simulink model "frt_only_up"  (R2012b)
settings: Solver=FixedStepDiscrete  SolverMode=SingleTasking  StartTime=0.0  StopTime=10000  RelTol=1e-3
undefined symbols (not defined in the file or in its folder): Down, Up
libraries: xbsIndex_r4 x5535, casper_library_misc x12, casper_library_communications x8, casper_library_scopes x2, xps_library x1
(part 8 of 48)

== system frt_only_up/trig1 ==
  synci : Inport
  adc_data : Inport  Port=2
  trig_pnt : Inport  Port=3
  Delay1 : xbsIndex_r4/Delay  rst=off  infoeditControl=Selection of Reset will increase slice count due to use of real FFs and instead of SRLs  en=off  latency=mult_latency+2  dbl_ovrd=off  reg_retiming=on  block_type=delay
      settings: block_version=11.4
  Delay2 : xbsIndex_r4/Delay  rst=off  infoeditControl=Selection of Reset will increase slice count due to use of real FFs and instead of SRLs  en=off  latency=mult_latency+2  dbl_ovrd=off  reg_retiming=on  block_type=delay
      settings: block_version=11.4
  Logical1 : xbsIndex_r4/Logical  logical_function=OR  inputs=4  en=off  latency=1  precision=Full  arith_type=Unsigned  n_bits=16  bin_pt=0  align_bp=on  dbl_ovrd=off  block_type=logical
  Mult : xbsIndex_r4/Mult  precision=Full  arith_type=Unsigned  n_bits=16  bin_pt=14  quantization=Truncate  overflow=Saturate  en=off  latency=mult_latency  dbl_ovrd=off  use_behavioral_HDL=on  opt=Speed  use_embedded=on  optimum_pipeline=off  pipeline=on  use_rpm=on  placement_style=Rectangular shape  block_type=mult
      settings: xl_area=[0, 0, 0, 0, 0, 0, 0]  block_version=10.1.3
  Reinterpret4 : xbsIndex_r4/Reinterpret  force_arith_type=on  arith_type="Signed  (2's comp)"  force_bin_pt=on  bin_pt=9  block_type=reinterpret
      settings: block_version=10.1.3
  Slice3 : xbsIndex_r4/Slice  nbits=10  boolean_output=off  mode=Lower Bit Location + Width  bit1=0  base1=MSB of Input  bit0=0  base0=LSB of Input  dbl_ovrd=off  block_type=slice
      settings: block_version=10.1.3
  Subsystem1 : Subsystem  mask{mult_latency=mult_latency}
      mask prompts: mult_latency "Multiplier latency"
  Subsystem2 : Subsystem  mask{mult_latency=mult_latency}
      mask prompts: mult_latency "Multiplier latency"
  Subsystem3 : Subsystem  mask{mult_latency=mult_latency}
      mask prompts: mult_latency "Multiplier latency"
  Subsystem5 : Subsystem  mask{mult_latency=mult_latency}
      mask prompts: mult_latency "Multiplier latency"
  bus_expand : Subsystem  AncestorBlock=casper_library_flow_control/bus_expand  mask(bus_expand){mode=divisions of equal size, outputNum=4, outputWidth=10, outputBinaryPt=9, outputArithmeticType=1, show_format=off, outputToWorkspace=off, variablePrefix=out, outputToModelAsWell=on}
      mask prompts: outputNum "Number of outputs:"; outputWidth "Output width:"; outputBinaryPt "Output binary point position:"; outputArithmeticType "Output arithmetic type (ufix=0, fix=1, bool=2):"; show_format "Print format string?"; outputToWorkspace "Output to workspace?"; variablePrefix "Variable name prefix:"; outputToModelAsWell "Output to model as well?"
      mask help:
      | Expands a 'bus' made using a bus_create or Xilinx
      | concat block.
      | The input will be divided into the specified number
      | of outputs with the specified arithmetic types.
      | Divisions are made from most significant bit.
      mask init: same as frt_only_up/bus_expand2
      settings: AttributesFormatString=4 outputs
      mask TypeOptions mode: divisions of equal size | divisions of arbitrary size
      mask Callback mode: bus_expand_callback();
      mask Callback outputWidth: bus_expand_callback();
      mask Callback outputToWorkspace: bus_expand_callback();
  synco : Outport
  data : Outport  Port=2
  trig : Outport  Port=3
  wires:
  bus_expand/4(lsb_out1) -> Subsystem3/1(din)
  bus_expand/3(out2) -> Subsystem2/1(din)
  bus_expand/2(out3) -> Subsystem1/1(din)
  bus_expand/1(msb_out4) -> Subsystem5/1(din)
  Delay1/1 -> data/1
  trig_pnt/1 -> Slice3/1
  Slice3/1 -> Reinterpret4/1
  Reinterpret4/1 -> Mult/2, Mult/1
  Mult/1 -> Subsystem3/2(thresh), Subsystem2/2(thresh), Subsystem1/2(thresh), Subsystem5/2(thresh)
  Logical1/1 -> trig/1
  adc_data/1 -> bus_expand/1(bus_in), Delay1/1
  Subsystem3/1(trig) -> Logical1/4
  Subsystem2/1(trig) -> Logical1/3
  Subsystem1/1(trig) -> Logical1/2
  Subsystem5/1(trig) -> Logical1/1
  synci/1 -> Delay2/1
  Delay2/1 -> synco/1

== system frt_only_up/trigger_level ==
  sim_1 : Inport
  frt_only_up_trigger_level_user_data_out : xbsIndex_r4/Gateway In  gui_display_data_type=Fixed-point  arith_type=Unsigned  n_bits=32  bin_pt=0  preci_type=Single  exp_width=8  frac_width=24  quantization="Round  (unbiased: +/- Inf)"  overflow=Saturate  period=1  dbl_ovrd=off  timing_constraint=None  locs_specified=off  LOCs={}  UseAsADC=off  ADCChannel='1'  inherit_from_input=off  hdl_port=on  block_type=gatewayin
  io_delay : xbsIndex_r4/Delay  rst=off  infoeditControl=Selection of Reset will increase slice count due to use of real FFs and instead of SRLs  en=off  latency=0  dbl_ovrd=off  reg_retiming=on  block_type=delay
  reint1 : xbsIndex_r4/Reinterpret  force_arith_type=on  arith_type=Unsigned  force_bin_pt=on  bin_pt=0  block_type=reinterpret
  slice_trigger_level : xbsIndex_r4/Slice  nbits=32  boolean_output=off  mode=Lower Bit Location + Width  bit1=0  base1=MSB of Input  bit0=0  base0=LSB of Input  dbl_ovrd=off  block_type=slice
  in_trigger_level : Outport
  wires:
  frt_only_up_trigger_level_user_data_out/1 -> io_delay/1
  sim_1/1 -> frt_only_up_trigger_level_user_data_out/1
  io_delay/1 -> slice_trigger_level/1
  slice_trigger_level/1 -> reint1/1
  reint1/1 -> in_trigger_level/1

== system frt_only_up/tx_metadata ==
  sim_1 : Inport
  sim_2 : Inport  Port=2
  convert1_1 : DataTypeConversion  OutDataTypeStr=fixdt('ufix16_En0')  LockScale=on
  convert1_2 : DataTypeConversion  OutDataTypeStr=fixdt('ufix16_En0')  LockScale=on
  convert2_1 : DataTypeConversion  OutDataTypeStr=fixdt('ufix16_En0')  ConvertRealWorld=Stored Integer (SI)  LockScale=on
  convert2_2 : DataTypeConversion  OutDataTypeStr=fixdt('ufix16_En0')  ConvertRealWorld=Stored Integer (SI)  LockScale=on
  frt_only_up_tx_metadata_user_data_out : xbsIndex_r4/Gateway In  gui_display_data_type=Fixed-point  arith_type=Unsigned  n_bits=32  bin_pt=0  preci_type=Single  exp_width=8  frac_width=24  quantization="Round  (unbiased: +/- Inf)"  overflow=Saturate  period=1  dbl_ovrd=off  timing_constraint=None  locs_specified=off  LOCs={}  UseAsADC=off  ADCChannel='1'  inherit_from_input=off  hdl_port=on  block_type=gatewayin
  gain_1 : Gain  Gain=65536
  gain_2 : Gain
  io_delay : xbsIndex_r4/Delay  rst=off  infoeditControl=Selection of Reset will increase slice count due to use of real FFs and instead of SRLs  en=off  latency=0  dbl_ovrd=off  reg_retiming=on  block_type=delay
  reint1 : xbsIndex_r4/Reinterpret  force_arith_type=on  arith_type=Unsigned  force_bin_pt=on  bin_pt=0  block_type=reinterpret
  reint2 : xbsIndex_r4/Reinterpret  force_arith_type=on  arith_type=Unsigned  force_bin_pt=on  bin_pt=0  block_type=reinterpret
  sim_add : Sum  OutDataTypeStr=uint32
  slice_board_id : xbsIndex_r4/Slice  nbits=16  boolean_output=off  mode=Lower Bit Location + Width  bit1=0  base1=MSB of Input  bit0=0  base0=LSB of Input  dbl_ovrd=off  block_type=slice
  slice_porttx : xbsIndex_r4/Slice  nbits=16  boolean_output=off  mode=Lower Bit Location + Width  bit1=0  base1=MSB of Input  bit0=16  base0=LSB of Input  dbl_ovrd=off  block_type=slice
  in_porttx : Outport
  in_board_id : Outport  Port=2
  wires:
  frt_only_up_tx_metadata_user_data_out/1 -> io_delay/1
  sim_add/1 -> frt_only_up_tx_metadata_user_data_out/1
  sim_1/1 -> convert1_1/1
  convert1_1/1 -> convert2_1/1
  convert2_1/1 -> gain_1/1
  gain_1/1 -> sim_add/1
  io_delay/1 -> slice_porttx/1, slice_board_id/1
  slice_porttx/1 -> reint1/1
  reint1/1 -> in_porttx/1
  sim_2/1 -> convert1_2/1
  convert1_2/1 -> convert2_2/1
  convert2_2/1 -> gain_2/1
  gain_2/1 -> sim_add/2
  slice_board_id/1 -> reint2/1
  reint2/1 -> in_board_id/1

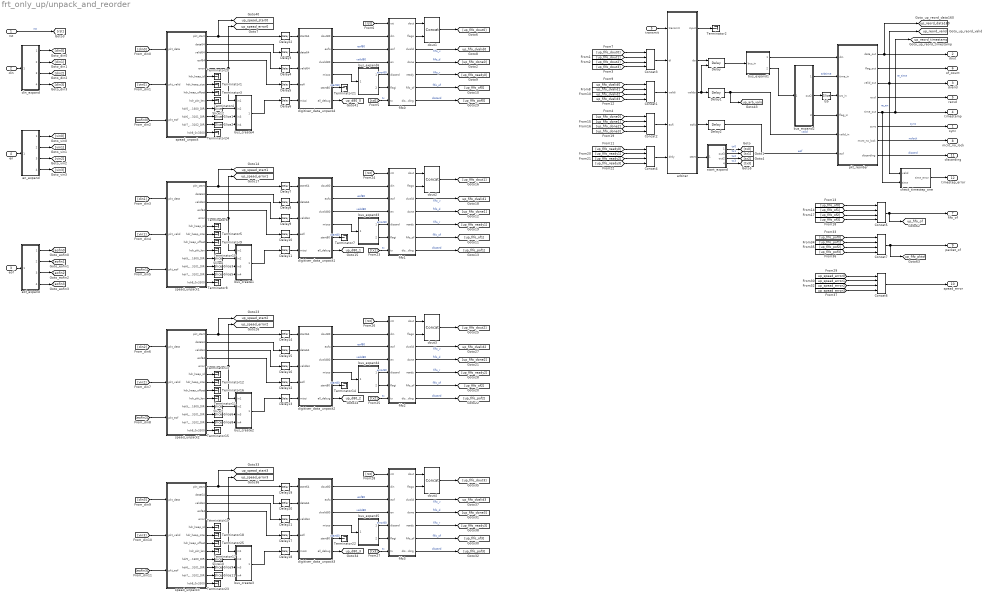
== system frt_only_up/unpack_and_reorder ==
  rst : Inport
  din : Inport  Port=2
  eof : Inport  Port=3
  en : Inport  Port=4
  transmit : Inport  Port=5
  Concat{1..7} (7 alike) : xbsIndex_r4/Concat  num_inputs=4  dbl_ovrd=off  block_type=concat
  Delay : xbsIndex_r4/Delay  rst=off  infoeditControl=Selection of Reset will increase slice count due to use of real FFs and instead of SRLs  en=on  latency=1  dbl_ovrd=off  reg_retiming=on  block_type=delay
  Delay{1..22} (22 alike) : xbsIndex_r4/Delay  rst=off  infoeditControl=Selection of Reset will increase slice count due to use of real FFs and instead of SRLs  en=off  latency=1  dbl_ovrd=off  reg_retiming=on  block_type=delay
      Delay10 settings: block_version=11.4
      Delay11 settings: block_version=11.4
      Delay12 settings: block_version=11.4
      Delay13 settings: block_version=11.4
      Delay14 settings: block_version=11.4
      Delay15 settings: block_version=11.4
      Delay16 settings: block_version=11.4
      Delay17 settings: block_version=11.4
      Delay18 settings: block_version=11.4
      Delay19 settings: block_version=11.4
      Delay20 settings: block_version=11.4
      Delay21 settings: block_version=11.4
      Delay22 settings: block_version=11.4
      Delay3 settings: block_version=11.4
      Delay4 settings: block_version=11.4
      Delay5 settings: block_version=11.4
      Delay6 settings: block_version=11.4
      Delay7 settings: block_version=11.4
      Delay8 settings: block_version=11.4
      Delay9 settings: block_version=11.4
  Slice{1,3,6,9} (4 alike) : xbsIndex_r4/Slice  nbits=2  boolean_output=off  mode=Lower Bit Location + Width  bit1=0  base1=MSB of Input  bit0=0  base0=LSB of Input  dbl_ovrd=off  block_type=slice
  Slice{4,7,10,12} (4 alike) : xbsIndex_r4/Slice  nbits=48 - n_bits_timestep  boolean_output=off  mode=Upper Bit Location + Width  bit1=0  base1=MSB of Input  bit0=0  base0=LSB of Input  dbl_ovrd=off  block_type=slice
  Slice{2,5,8,11} (4 alike) : xbsIndex_r4/Slice  nbits=1  boolean_output=off  mode=Lower Bit Location + Width  bit1=0  base1=MSB of Input  bit0=0  base0=LSB of Input  dbl_ovrd=off  block_type=slice
  Terminator{1..25} (25 alike) : Terminator
  arbiter : Subsystem  mask{n_inputs=4, n_bits_input=160 + 48 - n_bits_timestep + 2 + 1, mux_latency=1}
      mask prompts: n_inputs "number of inputs"; n_bits_input "input bit widths"; mux_latency "mux latency"
      mask init:
      | set_param([gcb, '/eofi_mux'], ...
      |     'n_bits', 'ones(1, n_inputs)', ...
      |     'mux_latency', 'mux_latency', ...
      |     'cmplx', 'off', 'misc', 'off');
      | set_param([gcb, '/di_mux'], ...
      |     'n_bits', 'repmat(n_bits_input, 1, n_inputs)', ...
      |     'mux_latency', 'mux_latency', ...
      |     'cmplx', 'off', 'misc', 'off');
      | set_param([gcb, '/validi_mux'], ...
      |     'n_bits', 'ones(1, n_inputs)', ...
      |     'mux_latency', 'mux_latency', ...
      |     'cmplx', 'off', 'misc', 'off');
      | set_param([gcb, '/busy_edge_rep'], ...
      |     'replication', 'n_inputs', ...
      |     'misc', 'off');
  bus_create1 : Subsystem  AncestorBlock=casper_library_flow_control/bus_create  mask(bus_create){inputNum=4}
      mask prompts: inputNum "Number of inputs:"
      mask init:
      | bus_create_init(gcb,...
      |     'inputNum', inputNum);
  bus_create2 : Subsystem  AncestorBlock=casper_library_flow_control/bus_create  mask(bus_create){inputNum=4}
      mask prompts: inputNum "Number of inputs:"
      mask init:
      | bus_create_init(gcb,...
      |     'inputNum', inputNum);
  bus_create3 : Subsystem  AncestorBlock=casper_library_flow_control/bus_create  mask(bus_create){inputNum=4}
      mask prompts: inputNum "Number of inputs:"
      mask init:
      | bus_create_init(gcb,...
      |     'inputNum', inputNum);
  bus_create4 : Subsystem  AncestorBlock=casper_library_flow_control/bus_create  mask(bus_create){inputNum=4}
      mask prompts: inputNum "Number of inputs:"
      mask init:
      | bus_create_init(gcb,...
      |     'inputNum', inputNum);
  bus_expand1 : Subsystem  AncestorBlock=casper_library_flow_control/bus_expand  mask(bus_expand){mode=divisions of arbitrary size, outputNum=1, outputWidth=[160, sum([48 - n_bits_timestep, 2, 1])], outputBinaryPt=[0 0], outputArithmeticType=[0 0], show_format=off, outputToWorkspace=off, variablePrefix=out, outputToModelAsWell=on}
      mask prompts: outputNum "Number of outputs:"; outputWidth "Output width [msb ... lsb]:"; outputBinaryPt "Output binary point position [msb ... lsb]:"; outputArithmeticType "Output arithmetic type (ufix=0, fix=1, bool=2) [msb ... lsb]:"; show_format "Print format string?"; outputToWorkspace "Output to workspace?"; variablePrefix "Variable name prefix:"; outputToModelAsWell "Output to model as well?"
      mask help:
      | Expands a 'bus' made using a bus_create or Xilinx
      | concat block.
      | The input will be divided into the specified number
      | of outputs with the specified arithmetic types.
      | Divisions are made from most significant bit.
      mask init: same as frt_only_up/bus_expand2
      settings: AttributesFormatString=2 outputs
      mask TypeOptions mode: divisions of equal size | divisions of arbitrary size
      mask Callback mode: bus_expand_callback();
      mask Callback outputWidth: bus_expand_callback();
      mask Callback outputToWorkspace: bus_expand_callback();
  bus_expand2 : Subsystem  AncestorBlock=casper_library_flow_control/bus_expand  mask(bus_expand){mode=divisions of arbitrary size, outputNum=1, outputWidth=[48 - n_bits_timestep, 2, 1], outputBinaryPt=[0 0 0], outputArithmeticType=[0 0 0], show_format=off, outputToWorkspace=off, variablePrefix=out, outputToModelAsWell=on}
      mask prompts: outputNum "Number of outputs:"; outputWidth "Output width [msb ... lsb]:"; outputBinaryPt "Output binary point position [msb ... lsb]:"; outputArithmeticType "Output arithmetic type (ufix=0, fix=1, bool=2) [msb ... lsb]:"; show_format "Print format string?"; outputToWorkspace "Output to workspace?"; variablePrefix "Variable name prefix:"; outputToModelAsWell "Output to model as well?"
      mask help:
      | Expands a 'bus' made using a bus_create or Xilinx
      | concat block.
      | The input will be divided into the specified number
      | of outputs with the specified arithmetic types.
      | Divisions are made from most significant bit.
      mask init: same as frt_only_up/bus_expand2
      settings: AttributesFormatString=3 outputs
      mask TypeOptions mode: divisions of equal size | divisions of arbitrary size
      mask Callback mode: bus_expand_callback();
      mask Callback outputWidth: bus_expand_callback();
      mask Callback outputToWorkspace: bus_expand_callback();
  bus_expand3 : Subsystem  AncestorBlock=casper_library_flow_control/bus_expand  mask(bus_expand){mode=divisions of arbitrary size, outputNum=1, outputWidth=[1, sum([48 - n_bits_timestep, 2, 1])], outputBinaryPt=[0 0], outputArithmeticType=[2 0], show_format=off, outputToWorkspace=off, variablePrefix=out, outputToModelAsWell=on}
      mask prompts: outputNum "Number of outputs:"; outputWidth "Output width [msb ... lsb]:"; outputBinaryPt "Output binary point position [msb ... lsb]:"; outputArithmeticType "Output arithmetic type (ufix=0, fix=1, bool=2) [msb ... lsb]:"; show_format "Print format string?"; outputToWorkspace "Output to workspace?"; variablePrefix "Variable name prefix:"; outputToModelAsWell "Output to model as well?"
      mask help:
      | Expands a 'bus' made using a bus_create or Xilinx
      | concat block.
      | The input will be divided into the specified number
      | of outputs with the specified arithmetic types.
      | Divisions are made from most significant bit.
      mask init: same as frt_only_up/bus_expand2
      settings: AttributesFormatString=2 outputs
      mask TypeOptions mode: divisions of equal size | divisions of arbitrary size
      mask Callback mode: bus_expand_callback();
      mask Callback outputWidth: bus_expand_callback();
      mask Callback outputToWorkspace: bus_expand_callback();
  bus_expand4 : Subsystem  AncestorBlock=casper_library_flow_control/bus_expand  mask(bus_expand){mode=divisions of arbitrary size, outputNum=1, outputWidth=[1, sum([48 - n_bits_timestep, 2, 1])], outputBinaryPt=[0 0], outputArithmeticType=[2 0], show_format=off, outputToWorkspace=off, variablePrefix=out, outputToModelAsWell=on}
      mask prompts: outputNum "Number of outputs:"; outputWidth "Output width [msb ... lsb]:"; outputBinaryPt "Output binary point position [msb ... lsb]:"; outputArithmeticType "Output arithmetic type (ufix=0, fix=1, bool=2) [msb ... lsb]:"; show_format "Print format string?"; outputToWorkspace "Output to workspace?"; variablePrefix "Variable name prefix:"; outputToModelAsWell "Output to model as well?"
      mask help:
      | Expands a 'bus' made using a bus_create or Xilinx
      | concat block.
      | The input will be divided into the specified number
      | of outputs with the specified arithmetic types.
      | Divisions are made from most significant bit.
      mask init: same as frt_only_up/bus_expand2
      settings: AttributesFormatString=2 outputs
      mask TypeOptions mode: divisions of equal size | divisions of arbitrary size
      mask Callback mode: bus_expand_callback();
      mask Callback outputWidth: bus_expand_callback();
      mask Callback outputToWorkspace: bus_expand_callback();
  bus_expand5 : Subsystem  AncestorBlock=casper_library_flow_control/bus_expand  mask(bus_expand){mode=divisions of arbitrary size, outputNum=1, outputWidth=[1, sum([48 - n_bits_timestep, 2, 1])], outputBinaryPt=[0 0], outputArithmeticType=[2 0], show_format=off, outputToWorkspace=off, variablePrefix=out, outputToModelAsWell=on}
      mask prompts: outputNum "Number of outputs:"; outputWidth "Output width [msb ... lsb]:"; outputBinaryPt "Output binary point position [msb ... lsb]:"; outputArithmeticType "Output arithmetic type (ufix=0, fix=1, bool=2) [msb ... lsb]:"; show_format "Print format string?"; outputToWorkspace "Output to workspace?"; variablePrefix "Variable name prefix:"; outputToModelAsWell "Output to model as well?"
      mask help:
      | Expands a 'bus' made using a bus_create or Xilinx
      | concat block.
      | The input will be divided into the specified number
      | of outputs with the specified arithmetic types.
      | Divisions are made from most significant bit.
      mask init: same as frt_only_up/bus_expand2
      settings: AttributesFormatString=2 outputs
      mask TypeOptions mode: divisions of equal size | divisions of arbitrary size
      mask Callback mode: bus_expand_callback();
      mask Callback outputWidth: bus_expand_callback();
      mask Callback outputToWorkspace: bus_expand_callback();
  bus_expand6 : Subsystem  AncestorBlock=casper_library_flow_control/bus_expand  mask(bus_expand){mode=divisions of arbitrary size, outputNum=1, outputWidth=[1, sum([48 - n_bits_timestep, 2, 1])], outputBinaryPt=[0 0], outputArithmeticType=[2 0], show_format=off, outputToWorkspace=off, variablePrefix=out, outputToModelAsWell=on}
      mask prompts: outputNum "Number of outputs:"; outputWidth "Output width [msb ... lsb]:"; outputBinaryPt "Output binary point position [msb ... lsb]:"; outputArithmeticType "Output arithmetic type (ufix=0, fix=1, bool=2) [msb ... lsb]:"; show_format "Print format string?"; outputToWorkspace "Output to workspace?"; variablePrefix "Variable name prefix:"; outputToModelAsWell "Output to model as well?"
      mask help:
      | Expands a 'bus' made using a bus_create or Xilinx
      | concat block.
      | The input will be divided into the specified number
      | of outputs with the specified arithmetic types.
      | Divisions are made from most significant bit.
      mask init: same as frt_only_up/bus_expand2
      settings: AttributesFormatString=2 outputs
      mask TypeOptions mode: divisions of equal size | divisions of arbitrary size
      mask Callback mode: bus_expand_callback();
      mask Callback outputWidth: bus_expand_callback();
      mask Callback outputToWorkspace: bus_expand_callback();
  check_timestep_one : Subsystem
  digitiser_data_unpack1 : Subsystem
  digitiser_data_unpack2 : Subsystem
  digitiser_data_unpack3 : Subsystem
  digitiser_data_unpack4 : Subsystem
  din_expand : Subsystem  AncestorBlock=casper_library_flow_control/bus_expand  mask(bus_expand){mode=divisions of equal size, outputNum=4, outputWidth=64, outputBinaryPt=0, outputArithmeticType=0, show_format=off, outputToWorkspace=off, variablePrefix=out, outputToModelAsWell=on}
      mask prompts: outputNum "Number of outputs:"; outputWidth "Output width:"; outputBinaryPt "Output binary point position:"; outputArithmeticType "Output arithmetic type (ufix=0, fix=1, bool=2):"; show_format "Print format string?"; outputToWorkspace "Output to workspace?"; variablePrefix "Variable name prefix:"; outputToModelAsWell "Output to model as well?"
      mask help:
      | Expands a 'bus' made using a bus_create or Xilinx
      | concat block.
      | The input will be divided into the specified number
      | of outputs with the specified arithmetic types.
      | Divisions are made from most significant bit.
      mask init: same as frt_only_up/bus_expand2
      settings: AttributesFormatString=4 outputs
      mask TypeOptions mode: divisions of equal size | divisions of arbitrary size
      mask Callback mode: bus_expand_callback();
      mask Callback outputWidth: bus_expand_callback();
      mask Callback outputToWorkspace: bus_expand_callback();
  dout{1..4} (4 alike) : xbsIndex_r4/Concat  num_inputs=2  dbl_ovrd=off  block_type=concat
  en_expand : Subsystem  AncestorBlock=casper_library_flow_control/bus_expand  mask(bus_expand){mode=divisions of equal size, outputNum=4, outputWidth=1, outputBinaryPt=0, outputArithmeticType=2, show_format=off, outputToWorkspace=off, variablePrefix=out, outputToModelAsWell=on}
      mask prompts: outputNum "Number of outputs:"; outputWidth "Output width:"; outputBinaryPt "Output binary point position:"; outputArithmeticType "Output arithmetic type (ufix=0, fix=1, bool=2):"; show_format "Print format string?"; outputToWorkspace "Output to workspace?"; variablePrefix "Variable name prefix:"; outputToModelAsWell "Output to model as well?"
      mask help:
      | Expands a 'bus' made using a bus_create or Xilinx
      | concat block.
      | The input will be divided into the specified number
      | of outputs with the specified arithmetic types.
      | Divisions are made from most significant bit.
      mask init: same as frt_only_up/bus_expand2
      settings: AttributesFormatString=4 outputs
      mask TypeOptions mode: divisions of equal size | divisions of arbitrary size
      mask Callback mode: bus_expand_callback();
      mask Callback outputWidth: bus_expand_callback();
      mask Callback outputToWorkspace: bus_expand_callback();
  eof_expand : Subsystem  AncestorBlock=casper_library_flow_control/bus_expand  mask(bus_expand){mode=divisions of equal size, outputNum=4, outputWidth=1, outputBinaryPt=0, outputArithmeticType=2, show_format=off, outputToWorkspace=off, variablePrefix=out, outputToModelAsWell=on}
      mask prompts: outputNum "Number of outputs:"; outputWidth "Output width:"; outputBinaryPt "Output binary point position:"; outputArithmeticType "Output arithmetic type (ufix=0, fix=1, bool=2):"; show_format "Print format string?"; outputToWorkspace "Output to workspace?"; variablePrefix "Variable name prefix:"; outputToModelAsWell "Output to model as well?"
      mask help:
      | Expands a 'bus' made using a bus_create or Xilinx
      | concat block.
      | The input will be divided into the specified number
      | of outputs with the specified arithmetic types.
      | Divisions are made from most significant bit.
      mask init: same as frt_only_up/bus_expand2
      settings: AttributesFormatString=4 outputs
      mask TypeOptions mode: divisions of equal size | divisions of arbitrary size
      mask Callback mode: bus_expand_callback();
      mask Callback outputWidth: bus_expand_callback();
      mask Callback outputToWorkspace: bus_expand_callback();
  fifo0 : Subsystem  mask{n_bits_din=80, scale_factor_bits=1, input_word_count_bits=n_bits_packet_size, n_bits_depth=n_bits_fifo_depth, n_bits_flag=sum([48 - n_bits_timestep, 2, 1]), bram_latency=bram_latency}
      mask prompts: n_bits_din "input data bit width"; scale_factor_bits "output width scale factor (2^? input bits)"; input_word_count_bits "max input word count (2^?)"; n_bits_depth "max buffer depth (2^? packets)"; n_bits_flag "flag bit width"; bram_latency "BRAM latency"
  fifo1 : Subsystem  mask{n_bits_din=80, scale_factor_bits=1, input_word_count_bits=n_bits_packet_size, n_bits_depth=n_bits_fifo_depth, n_bits_flag=sum([48 - n_bits_timestep, 2, 1]), bram_latency=bram_latency}
      mask prompts: n_bits_din "input data bit width"; scale_factor_bits "output width scale factor (2^? input bits)"; input_word_count_bits "max input word count (2^?)"; n_bits_depth "max buffer depth (2^? packets)"; n_bits_flag "flag bit width"; bram_latency "BRAM latency"
  fifo2 : Subsystem  mask{n_bits_din=80, scale_factor_bits=1, input_word_count_bits=n_bits_packet_size, n_bits_depth=n_bits_fifo_depth, n_bits_flag=sum([48 - n_bits_timestep, 2, 1]), bram_latency=bram_latency}
      mask prompts: n_bits_din "input data bit width"; scale_factor_bits "output width scale factor (2^? input bits)"; input_word_count_bits "max input word count (2^?)"; n_bits_depth "max buffer depth (2^? packets)"; n_bits_flag "flag bit width"; bram_latency "BRAM latency"
  fifo3 : Subsystem  mask{n_bits_din=80, scale_factor_bits=1, input_word_count_bits=n_bits_packet_size, n_bits_depth=n_bits_fifo_depth, n_bits_flag=sum([48 - n_bits_timestep, 2, 1]), bram_latency=bram_latency}
      mask prompts: n_bits_din "input data bit width"; scale_factor_bits "output width scale factor (2^? input bits)"; input_word_count_bits "max input word count (2^?)"; n_bits_depth "max buffer depth (2^? packets)"; n_bits_flag "flag bit width"; bram_latency "BRAM latency"
  lsb : xbsIndex_r4/Slice  nbits=1  boolean_output=off  mode=Lower Bit Location + Width  bit1=0  base1=MSB of Input  bit0=0  base0=LSB of Input  dbl_ovrd=off  block_type=slice
  pkt_reorder : Subsystem  mask{window_bits=n_bits_buffer_depth, window_size_bits=n_bits_packet_size - 1, n_bits_din=80, n_bits_flag=1, n_bits_timestamp=48}
      mask prompts: window_bits "Number of Windows to Buffer (2^?)"; window_size_bits "Window size (2^?)"; n_bits_din "Data bit width in"; n_bits_flag "Flag bit width in"; n_bits_timestamp "Timestamp bit width"
      mask init:
      | fmtstr = sprintf('Buffer space: 2^%i words', window_bits+window_size_bits);
      | set_param(gcb, 'AttributesFormatString', fmtstr);
      settings: AttributesFormatString=Buffer space: 2^11 words
  spead_unpack : Subsystem  Tag=casper:spead_unpack  AncestorBlock=casper_library_communications/spead_unpack  mask(spead_unpack_mask){max_pkt_len_bits=10, header_ids=0x1600, 0x3101, 0x3102, header_ind_ids=0x3300, spead_msw=64, spead_lsw=48, spead_version=4, combine_errors=on}
      mask prompts: max_pkt_len_bits "Max pkt length, 2^? 64-bit words"; header_ids "SPEAD direct header IDs (decimal)"; header_ind_ids "SPEAD indirect address IDs (decimal)"; spead_msw "SPEAD Flavour (MSw)"; spead_lsw "SPEAD Flavour (LSw)"; spead_version "SPEAD version"; combine_errors "Combine error flags"
      mask help: This block receives a 64-bit-word stream that contains a SPEAD stream. It checks the SPEAD headers are being correctly received. It presents the user with all headers on the first valid cycle of data along with a flag to indicate a header or packet-length error.
      mask init:
      | spead_unpack_init(gcb)
  spead_unpack1 : Subsystem  Tag=casper:spead_unpack  AncestorBlock=casper_library_communications/spead_unpack  mask(spead_unpack_mask){max_pkt_len_bits=10, header_ids=0x1600, 0x3101, 0x3102, header_ind_ids=0x3300, spead_msw=64, spead_lsw=48, spead_version=4, combine_errors=on}
      mask prompts: max_pkt_len_bits "Max pkt length, 2^? 64-bit words"; header_ids "SPEAD direct header IDs (decimal)"; header_ind_ids "SPEAD indirect address IDs (decimal)"; spead_msw "SPEAD Flavour (MSw)"; spead_lsw "SPEAD Flavour (LSw)"; spead_version "SPEAD version"; combine_errors "Combine error flags"
      mask help: This block receives a 64-bit-word stream that contains a SPEAD stream. It checks the SPEAD headers are being correctly received. It presents the user with all headers on the first valid cycle of data along with a flag to indicate a header or packet-length error.
      mask init:
      | spead_unpack_init(gcb)
  spead_unpack2 : Subsystem  Tag=casper:spead_unpack  AncestorBlock=casper_library_communications/spead_unpack  mask(spead_unpack_mask){max_pkt_len_bits=10, header_ids=0x1600, 0x3101, 0x3102, header_ind_ids=0x3300, spead_msw=64, spead_lsw=48, spead_version=4, combine_errors=on}
      mask prompts: max_pkt_len_bits "Max pkt length, 2^? 64-bit words"; header_ids "SPEAD direct header IDs (decimal)"; header_ind_ids "SPEAD indirect address IDs (decimal)"; spead_msw "SPEAD Flavour (MSw)"; spead_lsw "SPEAD Flavour (LSw)"; spead_version "SPEAD version"; combine_errors "Combine error flags"
      mask help: This block receives a 64-bit-word stream that contains a SPEAD stream. It checks the SPEAD headers are being correctly received. It presents the user with all headers on the first valid cycle of data along with a flag to indicate a header or packet-length error.
      mask init:
      | spead_unpack_init(gcb)
  spead_unpack3 : Subsystem  Tag=casper:spead_unpack  AncestorBlock=casper_library_communications/spead_unpack  mask(spead_unpack_mask){max_pkt_len_bits=10, header_ids=0x1600, 0x3101, 0x3102, header_ind_ids=0x3300, spead_msw=64, spead_lsw=48, spead_version=4, combine_errors=on}
      mask prompts: max_pkt_len_bits "Max pkt length, 2^? 64-bit words"; header_ids "SPEAD direct header IDs (decimal)"; header_ind_ids "SPEAD indirect address IDs (decimal)"; spead_msw "SPEAD Flavour (MSw)"; spead_lsw "SPEAD Flavour (LSw)"; spead_version "SPEAD version"; combine_errors "Combine error flags"
      mask help: This block receives a 64-bit-word stream that contains a SPEAD stream. It checks the SPEAD headers are being correctly received. It presents the user with all headers on the first valid cycle of data along with a flag to indicate a header or packet-length error.
      mask init:
      | spead_unpack_init(gcb)
  start_expand : Subsystem  AncestorBlock=casper_library_flow_control/bus_expand  mask(bus_expand){mode=divisions of equal size, outputNum=4, outputWidth=1, outputBinaryPt=0, outputArithmeticType=2, show_format=off, outputToWorkspace=off, variablePrefix=out, outputToModelAsWell=on}
      mask prompts: outputNum "Number of outputs:"; outputWidth "Output width:"; outputBinaryPt "Output binary point position:"; outputArithmeticType "Output arithmetic type (ufix=0, fix=1, bool=2):"; show_format "Print format string?"; outputToWorkspace "Output to workspace?"; variablePrefix "Variable name prefix:"; outputToModelAsWell "Output to model as well?"
      mask help:
      | Expands a 'bus' made using a bus_create or Xilinx
      | concat block.
      | The input will be divided into the specified number
      | of outputs with the specified arithmetic types.
      | Divisions are made from most significant bit.
      mask init: same as frt_only_up/bus_expand2
      settings: AttributesFormatString=4 outputs
      mask TypeOptions mode: divisions of equal size | divisions of arbitrary size
      mask Callback mode: bus_expand_callback();
      mask Callback outputWidth: bus_expand_callback();
      mask Callback outputToWorkspace: bus_expand_callback();
  sync : Outport
  dout : Outport  Port=2
  dvalid : Outport  Port=3
  timestamp : Outport  Port=4
  recvd : Outport  Port=5
  of_count : Outport  Port=6
  fifo_of : Outport  Port=7
  mcnt_no_lock : Outport  Port=8
  packet_of : Outport  Port=9
  spead_error : Outport  Port=10
  discarding : Outport  Port=11
  timestep_error : Outport  Port=12
  tag scope: up_arb_valid=global, up_d80_0=global, up_d80_1=global, up_d80_2=global, up_d80_3=global, up_fifo_dvalid0=global, up_fifo_dvalid1=global, up_fifo_dvalid2=global, up_fifo_dvalid3=global, up_fifo_of=global, up_fifo_pktof=global, up_reord_data160=global, up_reord_timestamp=global, up_reord_valid=global, up_spead_error0=global, up_spead_error1=global, up_spead_error2=global, up_spead_error3=global, up_spead_start0=global, up_spead_start1=global, up_spead_start2=global, up_spead_start3=global
  wires:
  check_timestep_one/1(time_error) -> timestep_error/1
  digitiser_data_unpack4/6(all_debug) -> [up_d80_0]
  digitiser_data_unpack4/5(start80) -> Terminator21/1  "start80"
  Delay6/1 -> digitiser_data_unpack4/5(misci)
  Delay5/1 -> digitiser_data_unpack4/4(eofi)
  Delay3/1 -> digitiser_data_unpack4/2(data64)
  Delay22/1 -> digitiser_data_unpack4/1(start64)
  Delay4/1 -> digitiser_data_unpack4/3(valid64)
  spead_unpack/1(pkt_start) -> Delay22/1, [up_spead_start0]
  spead_unpack/2(data64) -> Delay3/1
  spead_unpack/3(valid64) -> Delay4/1
  spead_unpack/4(eof64) -> Delay5/1
  spead_unpack/5(error) -> [up_spead_error0], bus_create4/1(in1)
  bus_create4/1(bus_out) -> Delay6/1
  [rst] -> fifo0/1(rst)
  Slice1/1 -> bus_create4/3(in3)
  Slice2/1 -> bus_create4/4(in4)
  Slice12/1 -> bus_create4/2(in2)
  spead_unpack/10(hdr5_0x1600_DIR) -> Slice12/1
  spead_unpack/11(hdr6_0x3101_DIR) -> Slice1/1
  spead_unpack/12(hdr7_0x3102_DIR) -> Slice2/1
  [tx0] -> fifo0/7(tx)  "tx"
  bus_expand6/1(msb_out2) -> fifo0/5(discard)  "error80"
  bus_expand6/2(lsb_out1) -> fifo0/6(flagi)
  digitiser_data_unpack4/4(misco) -> bus_expand6/1(bus_in)
  digitiser_data_unpack4/1(dout80) -> fifo0/2(din)
  digitiser_data_unpack4/2(eofo) -> fifo0/3(eof)  "eof80"
  digitiser_data_unpack4/3(dvalid80) -> fifo0/4(en)  "valid80"
  spead_unpack/6(hdr_heap_id) -> Terminator20/1
  spead_unpack/7(hdr_heap_size) -> Terminator1/1
  spead_unpack/8(hdr_heap_offset) -> Terminator3/1
  spead_unpack/9(hdr_pkt_len) -> Terminator4/1
  pkt_reorder/4(rcvd) -> recvd/1
  pkt_reorder/6(sync) -> sync/1  "sync"
  fifo0/4(done) -> [up_fifo_done0]  "fifo_d"
  dout1/1 -> [up_fifo_dout0]
  fifo0/3(dvalid) -> [up_fifo_dvalid0]  "fifo_v"
  fifo0/5(ready) -> [up_fifo_ready0]  "fifo_r"
  fifo0/6(fifo_of) -> [up_fifo_of0]  "fifo_of"
  arbiter/5(start) -> start_expand/1(bus_in)
  Concat4/1 -> arbiter/5(drdy)
  Concat2/1 -> arbiter/4(eofi)
  Concat3/1 -> arbiter/2(di)
  Concat1/1 -> arbiter/3(validi)
  transmit/1 -> arbiter/1(transmit)
  start_expand/1(msb_out4) -> [tx0]  "tx0"
  start_expand/2(out3) -> [tx1]  "tx1"
  start_expand/3(out2) -> [tx2]  "tx2"
  start_expand/4(lsb_out1) -> [tx3]  "tx3"
  [up_fifo_done0] -> Concat2/1
  [up_fifo_done3] -> Concat2/4
  [up_fifo_done1] -> Concat2/2
  [up_fifo_done2] -> Concat2/3
  [up_fifo_dout0] -> Concat3/1
  [up_fifo_dout1] -> Concat3/2
  [up_fifo_dvalid0] -> Concat1/1
  [up_fifo_dvalid1] -> Concat1/2
  [up_fifo_ready0] -> Concat4/1
  [up_fifo_ready1] -> Concat4/2
  Concat5/1 -> fifo_of/1, [up_fifo_of]
  [up_fifo_dout2] -> Concat3/3
  [up_fifo_dout3] -> Concat3/4
  [up_fifo_dvalid2] -> Concat1/3
  [up_fifo_dvalid3] -> Concat1/4
  [up_fifo_ready2] -> Concat4/3
  [up_fifo_ready3] -> Concat4/4
  arbiter/1(input) -> Terminator2/1
  [up_fifo_of0] -> Concat5/1
  [up_fifo_of1] -> Concat5/2
  [up_fifo_of2] -> Concat5/3
  [up_fifo_of3] -> Concat5/4
  rst/1 -> [rst]  "rst"
  pkt_reorder/2(flag_out) -> of_count/1
  din/1 -> din_expand/1(bus_in)
  en/1 -> en_expand/1(bus_in)
  eof/1 -> eof_expand/1(bus_in)
  bus_expand1/1(msb_out2) -> pkt_reorder/1(din)
  bus_expand1/2(lsb_out1) -> bus_expand2/1(bus_in)
  bus_expand2/1(msb_out3) -> pkt_reorder/2(time_in)  "arbtime"
  bus_expand2/3(lsb_out1) -> pkt_reorder/4(flag_in)
  fifo0/1(dout) -> dout1/1
  fifo0/2(flago) -> dout1/2
  bus_expand2/2(out2) -> lsb/1
  lsb/1 -> pkt_reorder/3(src_in)
  arbiter/2(do) -> Delay/1
  arbiter/3(valido) -> Delay1/1, Delay/2
  arbiter/4(eofo) -> Delay2/1
  Delay/1 -> bus_expand1/1(bus_in)
  Delay1/1 -> pkt_reorder/5(valid_in), [up_arb_valid]  "valid"
  Delay2/1 -> pkt_reorder/6(eof)  "eof"
  pkt_reorder/7(mcnt_no_lock) -> mcnt_no_lock/1  "nolock"
  [up_spead_error0] -> Concat6/1
  [up_spead_error1] -> Concat6/2
  [up_spead_error2] -> Concat6/3
  [up_spead_error3] -> Concat6/4
  Concat6/1 -> spead_error/1
  fifo0/7(discading) -> [up_fifo_pof0]  "discard"
  [up_fifo_pof0] -> Concat7/1
  [up_fifo_pof1] -> Concat7/2
  [up_fifo_pof2] -> Concat7/3
  [up_fifo_pof3] -> Concat7/4
  Concat7/1 -> packet_of/1, [up_fifo_pktof]
  pkt_reorder/8(discarding) -> discarding/1  "discard"
  pkt_reorder/5(time_out) -> timestamp/1, [up_reord_timestamp], check_timestep_one/2(time)  "re_time"
  pkt_reorder/3(valid_out) -> dvalid/1, check_timestep_one/1(valid), [up_reord_valid]  "re_en"
  pkt_reorder/1(data_out) -> dout/1, [up_reord_data160]
  spead_unpack/13(hdr8_0x3300) -> Terminator24/1
  din_expand/1(msb_out4) -> [din0]
  din_expand/2(out3) -> [din1]
  din_expand/3(out2) -> [din2]
  din_expand/4(lsb_out1) -> [din3]
  [din0] -> spead_unpack/1(pkt_data)
  en_expand/1(msb_out4) -> [vin0]
  en_expand/2(out3) -> [vin1]
  en_expand/3(out2) -> [vin2]
  en_expand/4(lsb_out1) -> [vin3]
  eof_expand/1(msb_out4) -> [eofin0]
  eof_expand/2(out3) -> [eofin1]
  eof_expand/3(out2) -> [eofin2]
  eof_expand/4(lsb_out1) -> [eofin3]
  [vin0] -> spead_unpack/2(pkt_valid)
  [eofin0] -> spead_unpack/3(pkt_eof)
  digitiser_data_unpack1/6(all_debug) -> [up_d80_1]
  digitiser_data_unpack1/5(start80) -> Terminator7/1  "start80"
  Delay11/1 -> digitiser_data_unpack1/5(misci)
  Delay10/1 -> digitiser_data_unpack1/4(eofi)
  Delay8/1 -> digitiser_data_unpack1/2(data64)
  Delay7/1 -> digitiser_data_unpack1/1(start64)
  Delay9/1 -> digitiser_data_unpack1/3(valid64)
  spead_unpack1/1(pkt_start) -> [up_spead_start1], Delay7/1
  spead_unpack1/2(data64) -> Delay8/1
  spead_unpack1/3(valid64) -> Delay9/1
  spead_unpack1/4(eof64) -> Delay10/1
  spead_unpack1/5(error) -> bus_create1/1(in1), [up_spead_error1]
  bus_create1/1(bus_out) -> Delay11/1
  [rst] -> fifo1/1(rst)
  Slice3/1 -> bus_create1/3(in3)
  Slice5/1 -> bus_create1/4(in4)
  Slice4/1 -> bus_create1/2(in2)
  spead_unpack1/10(hdr5_0x1600_DIR) -> Slice4/1
  spead_unpack1/11(hdr6_0x3101_DIR) -> Slice3/1
  spead_unpack1/12(hdr7_0x3102_DIR) -> Slice5/1
  [tx1] -> fifo1/7(tx)  "tx"
  bus_expand3/1(msb_out2) -> fifo1/5(discard)  "error80"
  bus_expand3/2(lsb_out1) -> fifo1/6(flagi)
  digitiser_data_unpack1/4(misco) -> bus_expand3/1(bus_in)
  digitiser_data_unpack1/1(dout80) -> fifo1/2(din)
  digitiser_data_unpack1/2(eofo) -> fifo1/3(eof)  "eof80"
  digitiser_data_unpack1/3(dvalid80) -> fifo1/4(en)  "valid80"
  spead_unpack1/6(hdr_heap_id) -> Terminator6/1
  spead_unpack1/7(hdr_heap_size) -> Terminator5/1
  spead_unpack1/8(hdr_heap_offset) -> Terminator9/1
  spead_unpack1/9(hdr_pkt_len) -> Terminator10/1
  fifo1/4(done) -> [up_fifo_done1]  "fifo_d"
  dout2/1 -> [up_fifo_dout1]
  fifo1/3(dvalid) -> [up_fifo_dvalid1]  "fifo_v"
  fifo1/5(ready) -> [up_fifo_ready1]  "fifo_r"
  fifo1/6(fifo_of) -> [up_fifo_of1]  "fifo_of"
  fifo1/1(dout) -> dout2/1
  fifo1/2(flago) -> dout2/2
  fifo1/7(discading) -> [up_fifo_pof1]  "discard"
  spead_unpack1/13(hdr8_0x3300) -> Terminator8/1
  [din1] -> spead_unpack1/1(pkt_data)
  [vin1] -> spead_unpack1/2(pkt_valid)
  [eofin1] -> spead_unpack1/3(pkt_eof)
  digitiser_data_unpack2/6(all_debug) -> [up_d80_2]
  digitiser_data_unpack2/5(start80) -> Terminator14/1  "start80"
  Delay13/1 -> digitiser_data_unpack2/5(misci)
  Delay12/1 -> digitiser_data_unpack2/4(eofi)
  Delay15/1 -> digitiser_data_unpack2/2(data64)
  Delay14/1 -> digitiser_data_unpack2/1(start64)
  Delay16/1 -> digitiser_data_unpack2/3(valid64)
  spead_unpack2/1(pkt_start) -> Delay14/1, [up_spead_start2]
  spead_unpack2/2(data64) -> Delay15/1
  spead_unpack2/3(valid64) -> Delay16/1
  spead_unpack2/4(eof64) -> Delay12/1
  spead_unpack2/5(error) -> [up_spead_error2], bus_create2/1(in1)
  bus_create2/1(bus_out) -> Delay13/1
  [rst] -> fifo2/1(rst)
  Slice6/1 -> bus_create2/3(in3)
  Slice8/1 -> bus_create2/4(in4)
  Slice7/1 -> bus_create2/2(in2)
  spead_unpack2/10(hdr5_0x1600_DIR) -> Slice7/1
  spead_unpack2/11(hdr6_0x3101_DIR) -> Slice6/1
  spead_unpack2/12(hdr7_0x3102_DIR) -> Slice8/1
  [tx2] -> fifo2/7(tx)  "tx"
  bus_expand4/1(msb_out2) -> fifo2/5(discard)  "error80"
  bus_expand4/2(lsb_out1) -> fifo2/6(flagi)
  digitiser_data_unpack2/4(misco) -> bus_expand4/1(bus_in)
  digitiser_data_unpack2/1(dout80) -> fifo2/2(din)
  digitiser_data_unpack2/2(eofo) -> fifo2/3(eof)  "eof80"
  digitiser_data_unpack2/3(dvalid80) -> fifo2/4(en)  "valid80"
  spead_unpack2/6(hdr_heap_id) -> Terminator13/1
  spead_unpack2/7(hdr_heap_size) -> Terminator12/1
  spead_unpack2/8(hdr_heap_offset) -> Terminator16/1
  spead_unpack2/9(hdr_pkt_len) -> Terminator11/1
  fifo2/4(done) -> [up_fifo_done2]  "fifo_d"
  dout3/1 -> [up_fifo_dout2]
  fifo2/3(dvalid) -> [up_fifo_dvalid2]  "fifo_v"
  fifo2/5(ready) -> [up_fifo_ready2]  "fifo_r"
  fifo2/6(fifo_of) -> [up_fifo_of2]  "fifo_of"
  fifo2/1(dout) -> dout3/1
  fifo2/2(flago) -> dout3/2
  fifo2/7(discading) -> [up_fifo_pof2]  "discard"
  spead_unpack2/13(hdr8_0x3300) -> Terminator15/1
  [din2] -> spead_unpack2/1(pkt_data)
  [vin2] -> spead_unpack2/2(pkt_valid)
  [eofin2] -> spead_unpack2/3(pkt_eof)
  digitiser_data_unpack3/6(all_debug) -> [up_d80_3]
  digitiser_data_unpack3/5(start80) -> Terminator22/1  "start80"
  Delay18/1 -> digitiser_data_unpack3/5(misci)
  Delay17/1 -> digitiser_data_unpack3/4(eofi)
  Delay20/1 -> digitiser_data_unpack3/2(data64)
  Delay19/1 -> digitiser_data_unpack3/1(start64)
  Delay21/1 -> digitiser_data_unpack3/3(valid64)
  spead_unpack3/1(pkt_start) -> [up_spead_start3], Delay19/1
  spead_unpack3/2(data64) -> Delay20/1
  spead_unpack3/3(valid64) -> Delay21/1
  spead_unpack3/4(eof64) -> Delay17/1
  spead_unpack3/5(error) -> bus_create3/1(in1), [up_spead_error3]
  bus_create3/1(bus_out) -> Delay18/1
  [rst] -> fifo3/1(rst)
  Slice9/1 -> bus_create3/3(in3)
  Slice11/1 -> bus_create3/4(in4)
  Slice10/1 -> bus_create3/2(in2)
  spead_unpack3/10(hdr5_0x1600_DIR) -> Slice10/1
  spead_unpack3/11(hdr6_0x3101_DIR) -> Slice9/1
  spead_unpack3/12(hdr7_0x3102_DIR) -> Slice11/1
  [tx3] -> fifo3/7(tx)  "tx"
  bus_expand5/1(msb_out2) -> fifo3/5(discard)  "error80"
  bus_expand5/2(lsb_out1) -> fifo3/6(flagi)
  digitiser_data_unpack3/4(misco) -> bus_expand5/1(bus_in)
  digitiser_data_unpack3/1(dout80) -> fifo3/2(din)
  digitiser_data_unpack3/2(eofo) -> fifo3/3(eof)  "eof80"
  digitiser_data_unpack3/3(dvalid80) -> fifo3/4(en)  "valid80"
  spead_unpack3/6(hdr_heap_id) -> Terminator19/1
  spead_unpack3/7(hdr_heap_size) -> Terminator18/1
  spead_unpack3/8(hdr_heap_offset) -> Terminator25/1
  spead_unpack3/9(hdr_pkt_len) -> Terminator17/1
  fifo3/4(done) -> [up_fifo_done3]  "fifo_d"
  dout4/1 -> [up_fifo_dout3]
  fifo3/3(dvalid) -> [up_fifo_dvalid3]  "fifo_v"
  fifo3/5(ready) -> [up_fifo_ready3]  "fifo_r"
  fifo3/6(fifo_of) -> [up_fifo_of3]  "fifo_of"
  fifo3/1(dout) -> dout4/1
  fifo3/2(flago) -> dout4/2
  fifo3/7(discading) -> [up_fifo_pof3]  "discard"
  spead_unpack3/13(hdr8_0x3300) -> Terminator23/1
  [din3] -> spead_unpack3/1(pkt_data)
  [vin3] -> spead_unpack3/2(pkt_valid)
  [eofin3] -> spead_unpack3/3(pkt_eof)
